simulink model "ejercicio1"  (Simulink 5.0)
settings: Solver=ode45  StartTime=0.0  StopTime=40  RelTol=1e-3
libraries: simulink_extras x1
settings Model: LastModifiedBy=-

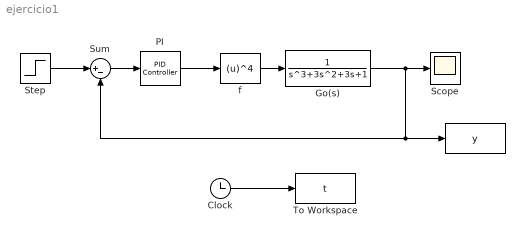
== system ejercicio1 ==
  " " : ToWorkspace  VariableName=y  SampleTime=0.01  SaveFormat=Array
      settings: Decimation=10
  Clock : Clock
      settings: Decimation=10
  Go(s) : TransferFcn  Denominator=[1 3 3 1]
  "PI " : simulink_extras/Additional Linear/PID Controller  P=0.15  I=0.15  D=0
  Scope : Scope
  Step : Step  Time=0  After=5.1  SampleTime=0
  Sum : Sum  Inputs=|+-  SaturateOnIntegerOverflow=on
  To Workspace : ToWorkspace  VariableName=t  SampleTime=0.01  SaveFormat=Array
      settings: Decimation=10
  f : Fcn  Expr=(u)^4
  wires:
  Step/1 -> Sum/1
  Go(s)/1 -> Scope/1, Sum/2, " "/1
  "PI "/1 -> f/1
  f/1 -> Go(s)/1
  Sum/1 -> "PI "/1
  Clock/1 -> To Workspace/1
